simulink subsystem "Wipers_OutputAquisition"  (R2025b)
settings: Solver=VariableStepAuto  StartTime=0.0  StopTime=10.0  RelTol=1e-3
libraries: simulink x7
settings Model: Creator=Sai Krishna  LastModifiedBy=Sai Krishna

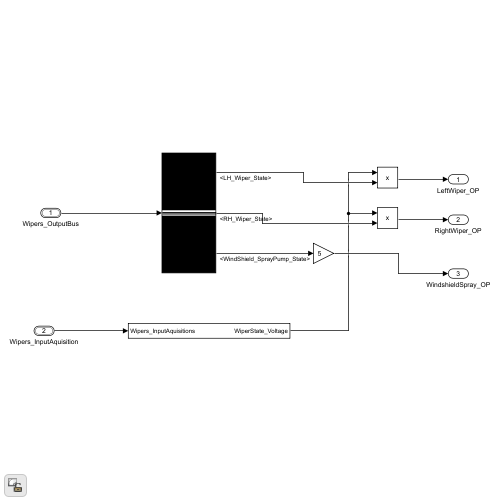
[thumbnail: Simulink's stored preview of the top-level diagram]
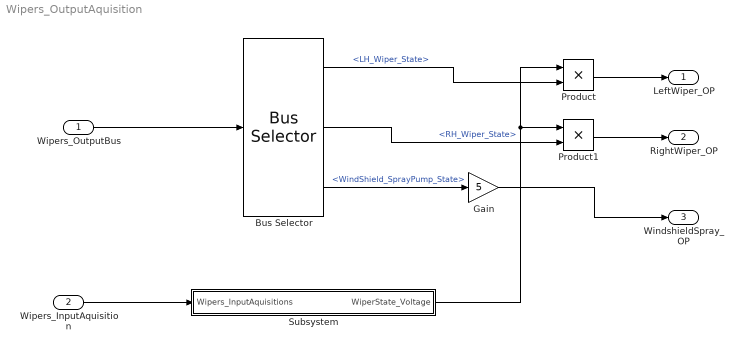
== system Wipers_OutputAquisition ==
  Wipers_OutputBus : Inport  OutDataTypeStr=Bus: Wipers_OutputBus
  Wipers_InputAquisition : Inport  Port=2  OutDataTypeStr=Bus: Wipers_InputBus
  Bus Selector : BusSelector  OutputSignals=LH_Wiper_State,RH_Wiper_State,WindShield_SprayPump_State
  Gain : Gain  Gain=5  OutDataTypeStr=double
  Product : Product  OutDataTypeStr=double
  Product1 : Product  OutDataTypeStr=double
  Subsystem : Subsystem
  LeftWiper_OP : Outport  OutDataTypeStr=double
  RightWiper_OP : Outport  Port=2  OutDataTypeStr=double
  WindshieldSpray_OP : Outport  Port=3  OutDataTypeStr=double
  wires:
  Wipers_OutputBus/1 -> Bus Selector/1
  Bus Selector/1 -> Product/2  "<LH_Wiper_State>"
  Bus Selector/2 -> Product1/2  "<RH_Wiper_State>"
  Bus Selector/3 -> Gain/1  "<WindShield_SprayPump_State>"
  Wipers_InputAquisition/1 -> Subsystem/1(Wipers_InputAquisitions)
  Subsystem/1(WiperState_Voltage) -> Product1/1, Product/1
  Product1/1 -> RightWiper_OP/1
  Product/1 -> LeftWiper_OP/1
  Gain/1 -> WindshieldSpray_OP/1

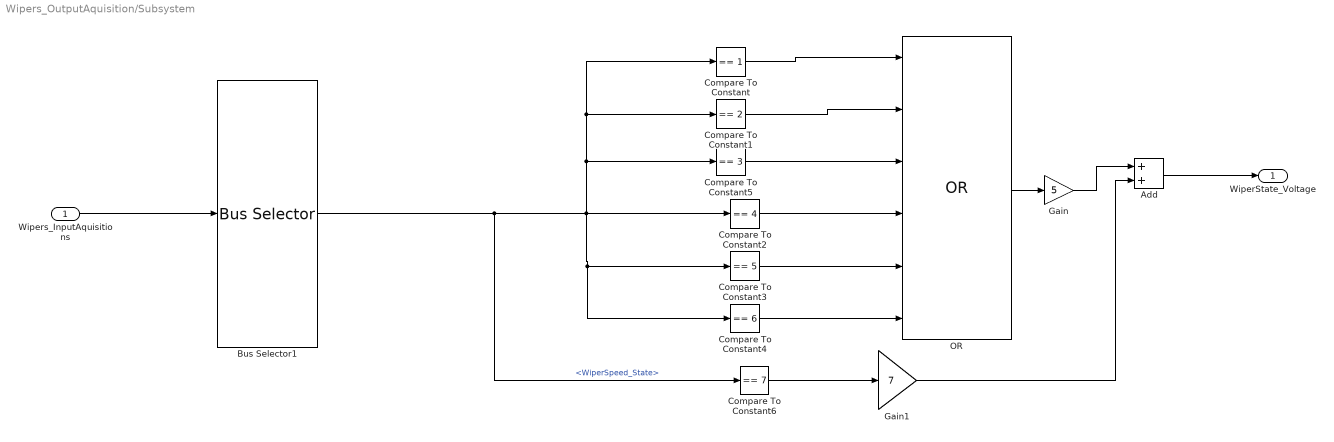
== system Wipers_OutputAquisition/Subsystem ==
  Wipers_InputAquisitions : Inport  OutDataTypeStr=Bus: Wipers_InputBus
  Add : Sum
  Bus Selector1 : BusSelector  OutputSignals=WiperSpeed_State
  Compare To Constant : simulink/Logic and Bit Operations/Compare To Constant  relop===  const=1  OutDataTypeStr=boolean
  Compare To Constant1 : simulink/Logic and Bit Operations/Compare To Constant  relop===  const=2  OutDataTypeStr=boolean
  Compare To Constant2 : simulink/Logic and Bit Operations/Compare To Constant  relop===  const=4  OutDataTypeStr=boolean
  Compare To Constant3 : simulink/Logic and Bit Operations/Compare To Constant  relop===  const=5  OutDataTypeStr=boolean
  Compare To Constant4 : simulink/Logic and Bit Operations/Compare To Constant  relop===  const=6  OutDataTypeStr=boolean
  Compare To Constant5 : simulink/Logic and Bit Operations/Compare To Constant  relop===  const=3  OutDataTypeStr=boolean
  Compare To Constant6 : simulink/Logic and Bit Operations/Compare To Constant  relop===  const=7  OutDataTypeStr=boolean
  Gain : Gain  Gain=5  OutDataTypeStr=double
  Gain1 : Gain  Gain=7  OutDataTypeStr=double
  OR : Logic  Operator=OR  Inputs=6  AllPortsSameDT=off  OutDataTypeStr=boolean
  WiperState_Voltage : Outport
  wires:
  Add/1 -> WiperState_Voltage/1
  OR/1 -> Gain/1
  Gain1/1 -> Add/2
  Compare To Constant4/1 -> OR/6
  Compare To Constant2/1 -> OR/4
  Compare To Constant/1 -> OR/1
  Wipers_InputAquisitions/1 -> Bus Selector1/1
  Compare To Constant6/1 -> Gain1/1
  Compare To Constant1/1 -> OR/2
  Gain/1 -> Add/1
  Compare To Constant5/1 -> OR/3
  Compare To Constant3/1 -> OR/5
  Bus Selector1/1 -> Compare To Constant2/1, Compare To Constant3/1, Compare To Constant4/1, Compare To Constant5/1, Compare To Constant1/1, Compare To Constant/1, Compare To Constant6/1  "<WiperSpeed_State>"
